simulink model "TestModel_simple"  (R2022b)
settings: Solver=VariableStepAuto  StartTime=0.0  StopTime=60  RelTol=1e-3
libraries: VACLib x3, simulink x1
settings Model: Creator=KarlO  LastModifiedBy=KarlO

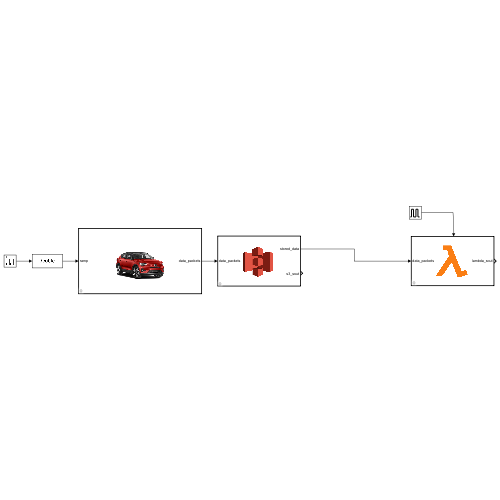
[thumbnail: Simulink's stored preview of the top-level diagram]
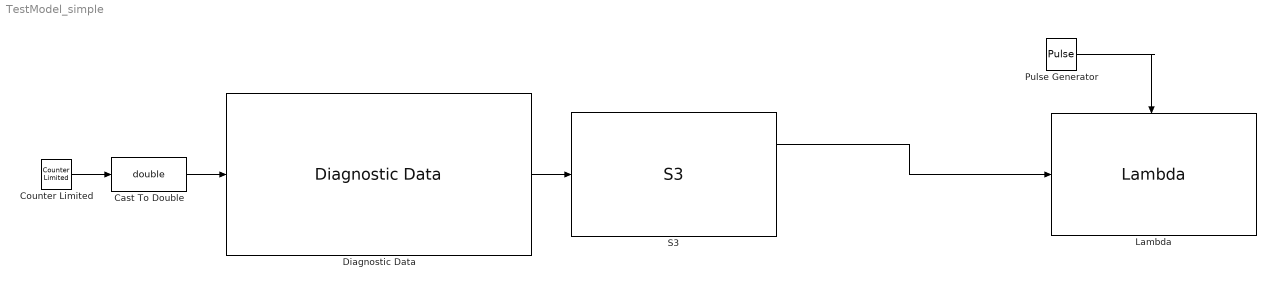
== system TestModel_simple ==
  Cast To Double : DataTypeConversion  OutDataTypeStr=double  SaturateOnIntegerOverflow=off  RndMeth=Floor
  Counter Limited : simulink/Sources/Counter Limited  uplimit=10  tsamp=1
  Diagnostic Data : VACLib/Vehicle Components/Diagnostic Data  cache_size=8  total_data_size=5000  spurts=10
      settings: LibrarySourceBlock=|
      | simulink/User-Defined
      | Functions/MATLAB Function
  Lambda : VACLib/AWS Components/Lambda  parallel_instances=600  lambda_chunk_size=300
      settings: LibrarySourceBlock=|
      | simulink/User-Defined
      | Functions/MATLAB Function
  Pulse Generator : DiscretePulseGenerator  PulseType=Time based  Period=0.2  PulseWidth=5
  S3 : VACLib/AWS Components/S3
      settings: LibrarySourceBlock=|
      | simulink/User-Defined
      | Functions/MATLAB Function
  wires:
  Counter Limited/1 -> Cast To Double/1
  Pulse Generator/1 -> Lambda/Trigger
  Cast To Double/1 -> Diagnostic Data/1
  Diagnostic Data/1 -> S3/1
  S3/1 -> Lambda/1
